simulink model "RADAR_System"  (R2019b)
settings: Solver=VariableStepAuto  StartTime=0.0  StopTime=stopTime  RelTol=1e-3
values from neighbouring files (symbols this model uses):
  indexToMeter = radar_dis_data(1, 2) - radar_dis_data(1, 1)    [RADAR_simulator.m]
libraries: dspstat3 x4
settings Model: Creator=ryoga  LastModifiedBy=ryoga

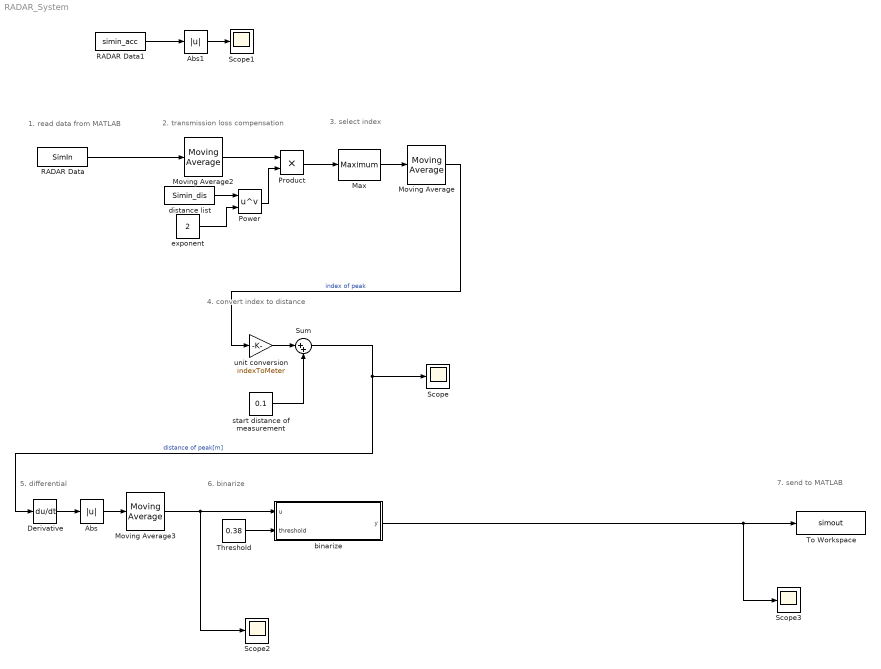
== system RADAR_System ==
  note: 7. send to MATLAB
  note: 6. binarize
  note: 5. differential
  note: 4. convert index to distance
  note: 3. select index
  note: 2. transmission loss compensation
  note: 1. read data from MATLAB
  Abs : Abs
  Abs1 : Abs
  Derivative : Derivative
  "Max " : dspstat3/Maximum  operation=maximum  fcn=Index  indexBase=One  operateOver=Each column  Dimension=1  InputProcessing=Columns as channels (frame based)  reset=None  roiEnable=off  roiType=Rectangles  roiPortion=Entire ROI  roiOutput=Individual statistics for each ROI  roiFlag=off  roundingMode=Floor  overflowMode=off  accumDataTypeStr=Inherit: Same as product output  accumLastDataTypeStr=Inherit: Same as product output
  Moving Average : dspstat3/Moving Average  Method=Sliding window  ForgettingFactorPort=off  SpecifyWindowLength=on  WindowLength=4  ForgettingFactor=0.9  SimulateUsing=Code generation
  Moving Average2 : dspstat3/Moving Average  Method=Sliding window  ForgettingFactorPort=off  SpecifyWindowLength=on  WindowLength=4  ForgettingFactor=0.9  SimulateUsing=Code generation
  Moving Average3 : dspstat3/Moving Average  Method=Sliding window  ForgettingFactorPort=off  SpecifyWindowLength=on  WindowLength=9  ForgettingFactor=0.9  SimulateUsing=Code generation
  Power : Math  Operator=pow  SignedPower=off  SaturateOnIntegerOverflow=on
  Product : Product
  RADAR Data : FromWorkspace  VariableName=SimIn  SampleTime=0.005  OutputAfterFinalValue=Setting to zero
  RADAR Data1 : FromWorkspace  VariableName=simin_acc  SampleTime=0.005  OutputAfterFinalValue=Setting to zero
  Scope{,1..3} (4 alike) : Scope
  Sum : Sum  Inputs=|++
  Threshold : Constant  Value=0.38
  To Workspace : ToWorkspace  VariableName=simout  SaveFormat=Timeseries  SampleTime=-1
  binarize : MATLAB Function  TreatAsAtomicUnit=on
  distance list : FromWorkspace  VariableName=Simin_dis  SampleTime=0.005  OutputAfterFinalValue=Setting to zero
  "exponent " : Constant  Value=2
  start distance of measurement : Constant  Value=0.1
  unit conversion : Gain  Gain=indexToMeter
  wires:
  unit conversion/1 -> Sum/1
  start distance of measurement/1 -> Sum/2
  Sum/1 -> Derivative/1, Scope/1  "distance of peak[m]"
  Threshold/1 -> binarize/2(threshold)
  Derivative/1 -> Abs/1
  Abs/1 -> Moving Average3/1
  RADAR Data/1 -> Moving Average2/1
  "Max "/1 -> Moving Average/1
  Moving Average/1 -> unit conversion/1  "index of peak"
  Moving Average3/1 -> Scope2/1, binarize/1(u)
  distance list/1 -> Power/1
  "exponent "/1 -> Power/2
  Power/1 -> Product/2
  Moving Average2/1 -> Product/1
  Product/1 -> "Max "/1
  Abs1/1 -> Scope1/1
  RADAR Data1/1 -> Abs1/1
  binarize/1(y) -> Scope3/1, To Workspace/1

== matlab function RADAR_System/binarize ==
  data: u input; y output; threshold input
function y = binarize(u, threshold)
    if u > threshold
        y = 1;
    else
        y = 0;
    end
